simulink subsystem "V4_Modell_Wagen"  (R2022b)
settings: Solver=VariableStepAuto  StartTime=0.0  StopTime=10.0  RelTol=1e-3
values from neighbouring files (symbols this model uses):
  A = 115.5    [V4_Parameter_Parameter_komplett_te.m]    (also in V4_Parameter_Wagen_Te.m = 0.01155; V4_Parameter_komplett.m = 0.01155)
  c_w = 0.81    [V4_Parameter_Parameter_komplett_te.m]    (also in V4_Parameter_Wagen_Te.m; V4_Parameter_komplett.m)
  Erdbeschleunigung = 9.81    [V4_Parameter_Parameter_komplett_te.m]    (also in V4_Parameter_Wagen_Te.m; V4_Parameter_komplett.m)
  k = (m_trans + m_Ersatz_Antr + m_Ersatz_Rad)./m_trans    [V4_Parameter_Parameter_komplett_te.m]    (also in V4_Parameter_Wagen_Te.m = 49.9140122158; V4_Parameter_komplett.m)
  m_ges = m_w + 4 * m_Rx    (= 1.7232)    [V4_Parameter_Parameter_komplett_te.m]    (also in V4_Parameter_Wagen_Te.m; V4_Parameter_komplett.m)
  m_trans = m_w + 4 * m_Rx    (= 1.7232)    [V4_Parameter_Parameter_komplett_te.m]    (also in V4_Parameter_Wagen_Te.m; V4_Parameter_komplett.m)
  mu = 0.1    [V4_Parameter_Parameter_komplett_te.m]    (also in V4_Parameter_Wagen_Te.m; V4_Parameter_komplett.m)
  phi_luft = 1.2    [V4_Parameter_Parameter_komplett_te.m]    (also in V4_Parameter_Wagen_Te.m; V4_Parameter_komplett.m)
settings Model: Creator=JSCHB  LastModifiedBy=Patrick

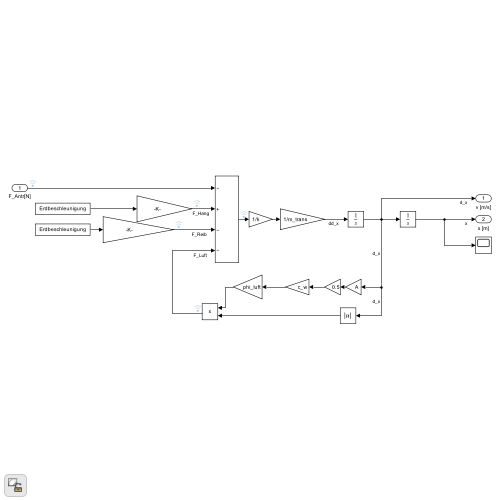
[thumbnail: Simulink's stored preview of the top-level diagram]
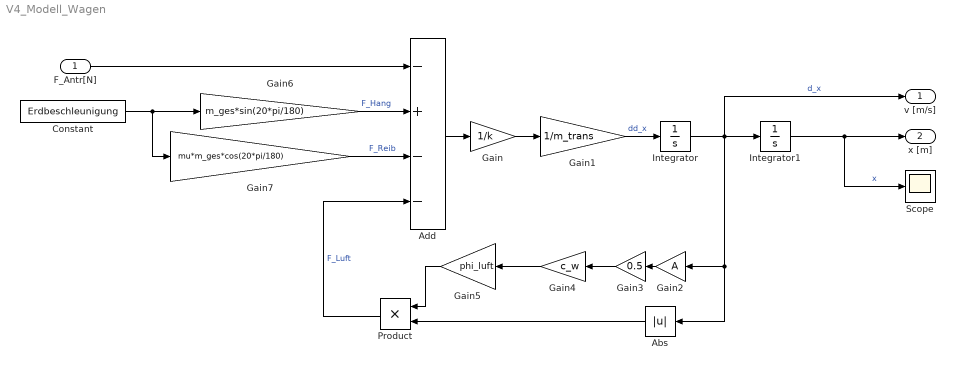
== system V4_Modell_Wagen ==
  F_Antr[N] : Inport
  Abs : Abs  SaturateOnIntegerOverflow=off
  Add : Sum  Inputs=-+--
  Constant : Constant  Value=Erdbeschleunigung
  Gain : Gain  Gain=1/k
  Gain1 : Gain  Gain=1/m_trans
  Gain2 : Gain  Gain=A
  Gain3 : Gain  Gain=0.5
  Gain4 : Gain  Gain=c_w
  Gain5 : Gain  Gain=phi_luft
  Gain6 : Gain  Gain=m_ges*sin(20*pi/180)
  Gain7 : Gain  Gain=mu*m_ges*cos(20*pi/180)
  Integrator : Integrator
  Integrator1 : Integrator
  Product : Product
  Scope : Scope
  v [m/s] : Outport
  x [m] : Outport  Port=2
  wires:
  Add/1 -> Gain/1
  Product/1 -> Add/4  "F_Luft"
  Gain5/1 -> Product/1
  Integrator1/1 -> x [m]/1, Scope/1  "x"
  Gain1/1 -> Integrator/1  "dd_x"
  Integrator/1 -> Integrator1/1, Abs/1, Gain2/1, v [m/s]/1  "d_x"
  Gain4/1 -> Gain5/1
  Abs/1 -> Product/2
  Gain3/1 -> Gain4/1
  Gain2/1 -> Gain3/1
  Gain/1 -> Gain1/1
  F_Antr[N]/1 -> Add/1
  Gain6/1 -> Add/2  "F_Hang"
  Constant/1 -> Gain6/1, Gain7/1
  Gain7/1 -> Add/3  "F_Reib"
